simulink model "copy2"  (R2019a)
settings: Solver=FixedStepAuto  StartTime=0.0  StopTime=inf  FixedStep=0.000001  RelTol=1e-3
libraries: dspstat3 x4, simulink x1
settings Model: NumberOfSteps=16  Creator=vardhah  LastModifiedBy=vardhah
settings DataIOCC: ReturnWorkspaceOutputs=off
settings DebuggingCC: UnderSpecifiedDimensionMsg=warning  ArithmeticOperatorsInVariantConditions=warning

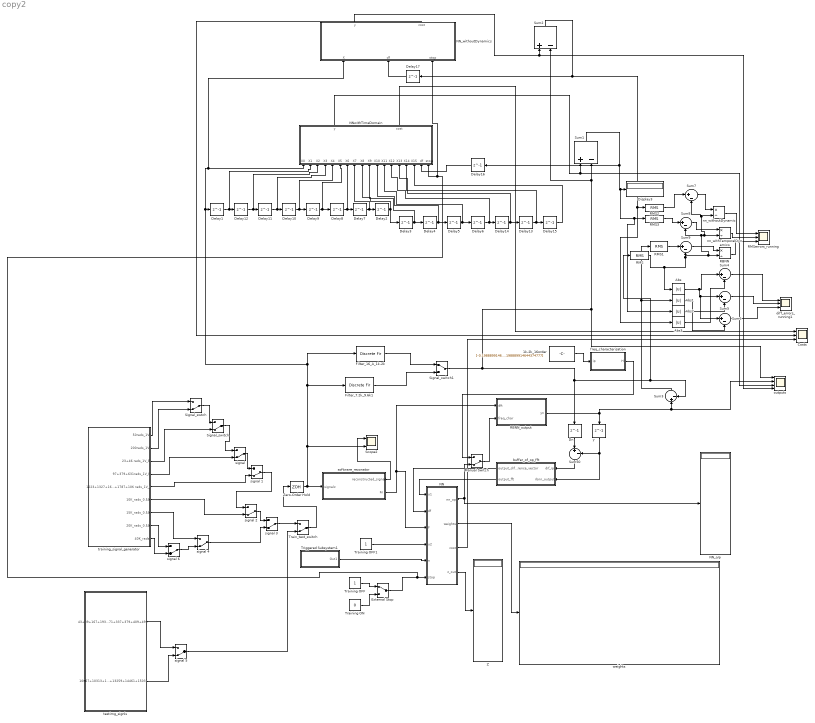
== system copy2 ==
  1k-2k_16order : Constant  Value=[-0.198889914644374777 0.0882189428518377339 0.0736891495871065116 0.0638368801789635787 0.0566372642221577294 0.0523172683654103132 0.0494565343907736044 0.048157521822162791 0.048157521822162791 0.0494565343907736044 0.0523172683654103132 0.0566372642221577294 0.0638368801789635787 0.0736891495871065116 0.0882189428518377339 -0.198889914644374777]  VectorParams1D=off
  Abs{,1..3} (4 alike) : Abs
  Costs : Scope  NumInputPorts=3
  Delay{1..17} (17 alike) : Delay  DelayLength=1  InitialCondition=0
  Display3 : Display
  Dn : Delay  DelayLength=1  InitialCondition=0
  External Stop : ManualSwitch
  Filter_16_A_1k-2k : DiscreteFir  Tag=BlockMethodSubSystem  Coefficients=[-0.198889914644374777 0.0882189428518377339 0.0736891495871065116 0.0638368801789635787 0.0566372642221577294 0.0523172683654103132 0.0494565343907736044 0.048157521822162791 0.048157521822162791 0.0494565343907736044 0.0523172683654103132 0.0566372642221577294 0.0638368801789635787 0.0736891495871065116 0.0882189428518377339 -0.198889914644374777]  InputProcessing=Columns as channels (frame based)
  Filter_7.2k_9.6k1 : DiscreteFir  Tag=BlockMethodSubSystem  Coefficients=[-0.0120785049852322399 -0.0942455273574688279 0.0101245004695954266 0.125460404555770566 0.034165372769331126 -0.1614987160724079 -0.0984930555982914957 0.150982315564688691 0.150982315564688691 -0.0984930555982914957 -0.1614987160724079 0.034165372769331126 0.125460404555770566 0.0101245004695954266 -0.0942455273574688279 -0.0120785049852322399]  InputProcessing=Columns as channels (frame based)
  Manual Switch : ManualSwitch  CurrentSetting=0  varsize=on
  NN : MATLAB Function  TreatAsAtomicUnit=on
  NN_o/p : Display
  NN_withoutDynamics : MATLAB Function  TreatAsAtomicUnit=on
  NNwithTimeDomain : MATLAB Function  TreatAsAtomicUnit=on
  RBNN : Product  Inputs=*/
  RBNN_output : MATLAB Function  TreatAsAtomicUnit=on
  RMS{,1..3} (4 alike) : dspstat3/RMS  run=on  directionMode=Each column  dimension=1  InputProcessing=Columns as channels (frame based)  reset_popup=None
  RMSerrors_running : Scope  NumInputPorts=3
  Scope2 : Scope  NumInputPorts=2
  Signal_switch : ManualSwitch  CurrentSetting=0
  Signal_switch1 : ManualSwitch
  Signal_swtch : ManualSwitch  CurrentSetting=0
  Sum1 : Sum  Inputs=+-
  Sum2 : Sum  Inputs=+-
  Sum{3..9,50} (8 alike) : Sum  Inputs=|+-
  Train_test_switch : ManualSwitch  CurrentSetting=0
  Training OFF : Constant
  Training OFF1 : Constant
  Training ON : Constant  Value=0
  Triggered Subsystem1 : Subsystem  TreatAsAtomicUnit=on
  Z : Display
  Zero-Order Hold : ZeroOrderHold  SampleTime=0.00001
  buffer_of_op_fft : MATLAB Function  TreatAsAtomicUnit=on
  diff_errors_running1 : Scope  NumInputPorts=3
  freq_characterisation : MATLAB Function  TreatAsAtomicUnit=on
  nn_withTemporalDynamics : Product  Inputs=*/
  nn_withoutDynamic : Product  Inputs=*/
  outputs : Scope  NumInputPorts=4
  signal {,1..6} (7 alike) : ManualSwitch  CurrentSetting=0
  software_rezonator : MATLAB Function  TreatAsAtomicUnit=on
  testimg_signls : Subsystem
  training_signal_generator : Subsystem
  weights : Display
  y : Delay  DelayLength=1  InitialCondition=0
  wires:
  software_rezonator/1(reconstructed_signal) -> Scope2/1
  software_rezonator/2(Fn) -> RBNN_output/1(dft), NN/3(F)
  RBNN_output/1(yn) -> Sum3/1, outputs/2, y/1
  Dn/1 -> Sum50/1
  y/1 -> buffer_of_op_fft/2(rbnn_output), Sum50/2
  Manual Switch/1 -> RBNN_output/2(freq_char)
  freq_characterisation/1(H) -> Manual Switch/1
  NN/1(nn_op) -> Manual Switch/2, NN_o/p/1
  External Stop/1 -> NN_withoutDynamics/3(stop), NNwithTimeDomain/18(stop), NN/6(stop)
  Training OFF/1 -> External Stop/1
  Training ON/1 -> External Stop/2
  NN/3(cost) -> Costs/3
  NN/2(weights) -> weights/1
  NN/4(z_out) -> Z/1
  1k-2k_16order/1 -> freq_characterisation/1(ip)
  Triggered Subsystem1/1(Out1) -> NN/5(n)
  Sum50/1 -> buffer_of_op_fft/1(dif_ip)
  buffer_of_op_fft/1(output_difference_vector) -> NN/2(df)
  buffer_of_op_fft/2(output_fft) -> NN/1(u1)
  Training OFF1/1 -> NN/4(u2)
  Signal_switch/1 -> "signal "/1
  Signal_swtch/1 -> Signal_switch/1
  "signal "/1 -> signal 1/1
  signal 1/1 -> signal 2/1
  training_signal_generator/4(97+379+631rads_1V_E) -> "signal "/2
  training_signal_generator/1(50rads_1V) -> Signal_swtch/1
  training_signal_generator/2(200rads_1V) -> Signal_swtch/2
  training_signal_generator/3(23+46 rads_1V_E) -> Signal_switch/2
  training_signal_generator/5(1223+1327+1637+1787+10K rads_1V_E) -> signal 1/2
  training_signal_generator/6(10K_rads_0.5A) -> signal 2/2
  signal 2/1 -> signal 3/1
  NNwithTimeDomain/1(y) -> outputs/3, Sum1/1
  Delay16/1 -> NNwithTimeDomain/17(df)
  Delay4/1 -> NNwithTimeDomain/11(X10), Delay5/1
  Delay6/1 -> Delay14/1, NNwithTimeDomain/13(X12)
  Delay5/1 -> NNwithTimeDomain/12(X11), Delay6/1
  NNwithTimeDomain/2(cost) -> Costs/1
  Delay2/1 -> Delay3/1, NNwithTimeDomain/9(X8)
  Delay15/1 -> NNwithTimeDomain/16(X15)
  Delay13/1 -> NNwithTimeDomain/15(X14), Delay15/1
  Delay14/1 -> NNwithTimeDomain/14(X13), Delay13/1
  Delay10/1 -> NNwithTimeDomain/5(X4), Delay9/1
  Zero-Order Hold/1 -> Scope2/2, Filter_16_A_1k-2k/1, NN_withoutDynamics/1(X), NNwithTimeDomain/1(X0), Delay1/1, Filter_7.2k_9.6k1/1, software_rezonator/1(signalz)
  Delay3/1 -> Delay4/1, NNwithTimeDomain/10(X9)
  Delay7/1 -> Delay2/1, NNwithTimeDomain/8(X7)
  Delay8/1 -> NNwithTimeDomain/7(X6), Delay7/1
  Delay1/1 -> NNwithTimeDomain/2(X1), Delay12/1
  Delay9/1 -> Delay8/1, NNwithTimeDomain/6(X5)
  Delay12/1 -> NNwithTimeDomain/3(X2), Delay11/1
  Delay11/1 -> Delay10/1, NNwithTimeDomain/4(X3)
  Sum1/1 -> Abs2/1, RMS3/1, Display3/1, Delay16/1
  NN_withoutDynamics/1(y) -> outputs/4, Sum2/1
  Delay17/1 -> NN_withoutDynamics/2(df)
  Sum2/1 -> Abs3/1, RMS2/1, Delay17/1
  NN_withoutDynamics/2(cost) -> Costs/2
  training_signal_generator/7(15K_rads_0.5A) -> signal 4/1
  signal 4/1 -> signal 3/2
  Filter_7.2k_9.6k1/1 -> Signal_switch1/2
  Filter_16_A_1k-2k/1 -> Signal_switch1/1
  Signal_switch1/1 -> Sum2/2, Sum1/2, outputs/1, RMS/1, Sum3/2, Dn/1
  nn_withoutDynamic/1 -> RMSerrors_running/1
  nn_withTemporalDynamics/1 -> RMSerrors_running/2
  RBNN/1 -> RMSerrors_running/3
  RMS/1 -> Sum7/2, nn_withoutDynamic/2, nn_withTemporalDynamics/2, Sum8/2, RBNN/2, Sum9/2, Abs/1
  Sum3/1 -> Abs1/1, RMS1/1
  Abs/1 -> Sum6/1, Sum5/1, Sum4/1
  Abs1/1 -> Sum6/2
  Abs3/1 -> Sum4/2
  Abs2/1 -> Sum5/2
  Sum4/1 -> diff_errors_running1/1
  Sum5/1 -> diff_errors_running1/2
  Sum6/1 -> diff_errors_running1/3
  RMS1/1 -> Sum9/1
  RMS3/1 -> Sum8/1
  Sum8/1 -> nn_withTemporalDynamics/1
  RMS2/1 -> Sum7/1
  Sum7/1 -> nn_withoutDynamic/1
  testimg_signls/1(43+89+167+193+229+271+337+379+409+499) -> signal 5/1
  testimg_signls/2("10067+10313+10987+11299+11491+12161+12451+13259+14461+15031 ") -> signal 5/2
  signal 3/1 -> Train_test_switch/1
  signal 5/1 -> Train_test_switch/2
  Train_test_switch/1 -> Zero-Order Hold/1
  signal 6/1 -> signal 4/2
  training_signal_generator/8(20K_rads_0.5A) -> signal 6/1
  training_signal_generator/9(40K_rads) -> signal 6/2
  Sum9/1 -> RBNN/1

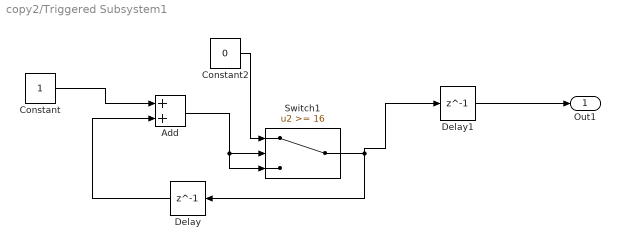
== system copy2/Triggered Subsystem1 ==
  Add : Sum
  Constant : Constant
  Constant2 : Constant  Value=0
  Delay : Delay  DelayLength=1  InitialCondition=0
  Delay1 : Delay  DelayLength=1  InitialCondition=0
  Switch1 : Switch  Threshold=16
  Out1 : Outport
  wires:
  Constant2/1 -> Switch1/1
  Constant/1 -> Add/1
  Switch1/1 -> Delay1/1, Delay/1
  Delay/1 -> Add/2
  Add/1 -> Switch1/3, Switch1/2
  Delay1/1 -> Out1/1

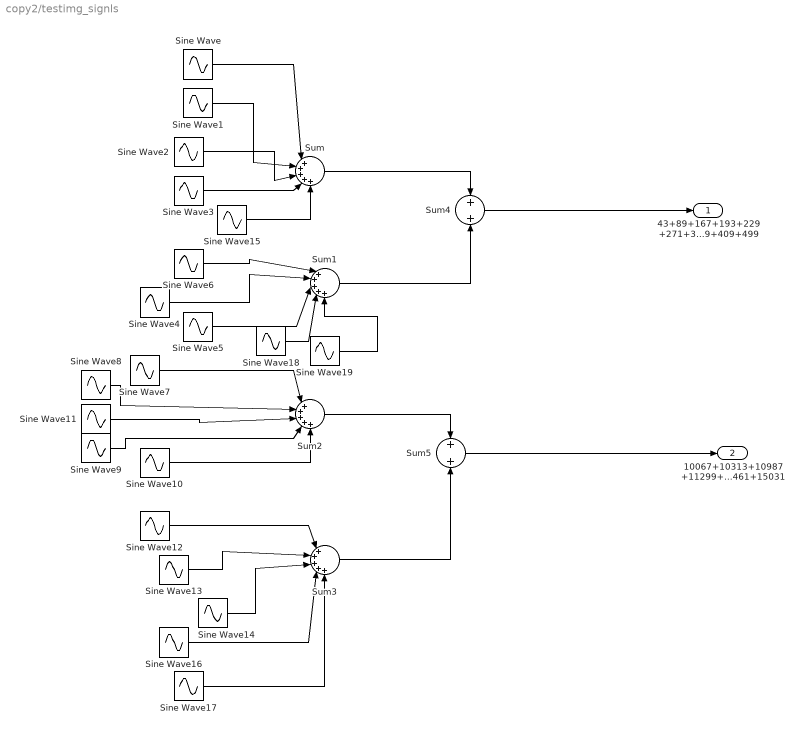
== system copy2/testimg_signls ==
  Sine Wave : Sin  Amplitude=0.1  Frequency=43  SampleTime=0
  Sine Wave1 : Sin  Amplitude=0.1  Frequency=89  SampleTime=0
  Sine Wave10 : Sin  Amplitude=0.1  Frequency=11491  SampleTime=0
  Sine Wave11 : Sin  Amplitude=0.1  Frequency=10987  SampleTime=0
  Sine Wave12 : Sin  Amplitude=0.1  Frequency=12161  SampleTime=0
  Sine Wave13 : Sin  Amplitude=0.1  Frequency=12451  SampleTime=0
  Sine Wave14 : Sin  Amplitude=0.1  Frequency=13259  SampleTime=0
  Sine Wave15 : Sin  Amplitude=0.1  Frequency=229  SampleTime=0
  Sine Wave16 : Sin  Amplitude=0.1  Frequency=14461  SampleTime=0
  Sine Wave17 : Sin  Amplitude=0.1  Frequency=15031  SampleTime=0
  Sine Wave18 : Sin  Amplitude=0.1  Frequency=409  SampleTime=0
  Sine Wave19 : Sin  Amplitude=0.1  Frequency=499  SampleTime=0
  Sine Wave2 : Sin  Amplitude=0.1  Frequency=167  SampleTime=0
  Sine Wave3 : Sin  Amplitude=0.1  Frequency=193  SampleTime=0
  Sine Wave4 : Sin  Amplitude=0.1  Frequency=337  SampleTime=0
  Sine Wave5 : Sin  Amplitude=0.1  Frequency=379  SampleTime=0
  Sine Wave6 : Sin  Amplitude=0.1  Frequency=271  SampleTime=0
  Sine Wave7 : Sin  Amplitude=0.1  Frequency=10067  SampleTime=0
  Sine Wave8 : Sin  Amplitude=0.1  Frequency=10313  SampleTime=0
  Sine Wave9 : Sin  Amplitude=0.1  Frequency=11299  SampleTime=0
  Sum{,1..3} (4 alike) : Sum  Inputs=|+++++
  Sum4 : Sum
  Sum5 : Sum
  43+89+167+193+229+271+337+379+409+499 : Outport
  "10067+10313+10987+11299+11491+12161+12451+13259+14461+15031 " : Outport  Port=2
  wires:
  Sine Wave4/1 -> Sum1/2
  Sine Wave5/1 -> Sum1/3
  Sine Wave6/1 -> Sum1/1
  Sine Wave7/1 -> Sum2/1
  Sine Wave8/1 -> Sum2/2
  Sine Wave11/1 -> Sum2/3
  Sine Wave9/1 -> Sum2/4
  Sine Wave10/1 -> Sum2/5
  Sine Wave/1 -> Sum/1
  Sine Wave1/1 -> Sum/2
  Sine Wave2/1 -> Sum/3
  Sine Wave3/1 -> Sum/4
  Sine Wave15/1 -> Sum/5
  Sine Wave17/1 -> Sum3/5
  Sine Wave16/1 -> Sum3/4
  Sine Wave14/1 -> Sum3/3
  Sine Wave13/1 -> Sum3/2
  Sine Wave12/1 -> Sum3/1
  Sine Wave18/1 -> Sum1/4
  Sine Wave19/1 -> Sum1/5
  Sum1/1 -> Sum4/2
  Sum/1 -> Sum4/1
  Sum4/1 -> 43+89+167+193+229+271+337+379+409+499/1
  Sum5/1 -> "10067+10313+10987+11299+11491+12161+12451+13259+14461+15031 "/1
  Sum2/1 -> Sum5/1
  Sum3/1 -> Sum5/2

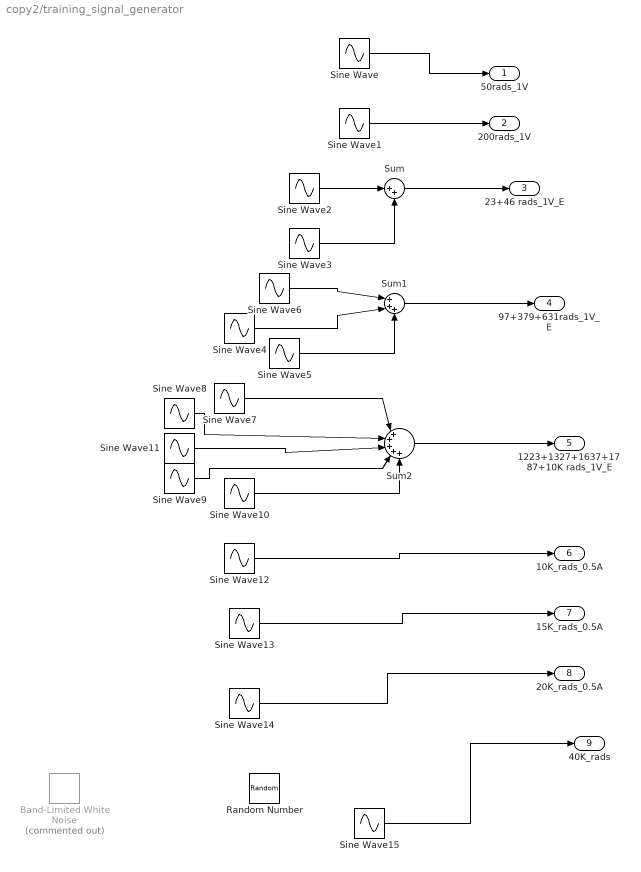
== system copy2/training_signal_generator ==
  Band-Limited White Noise : simulink/Sources/Band-Limited White Noise  Commented=on  Cov=[0.1]  Ts=0.1  seed=[23341]
  Random Number : RandomNumber  Variance=0.5  SampleTime=0.0001
  Sine Wave : Sin  Frequency=50  SampleTime=0
  Sine Wave1 : Sin  Frequency=200  SampleTime=0
  Sine Wave10 : Sin  Amplitude=0.2  Frequency=10000  SampleTime=0
  Sine Wave11 : Sin  Amplitude=0.2  Frequency=1637  SampleTime=0
  Sine Wave12 : Sin  Amplitude=0.5  Frequency=10000  SampleTime=0
  Sine Wave13 : Sin  Amplitude=0.5  Frequency=15000  SampleTime=0
  Sine Wave14 : Sin  Amplitude=0.5  Frequency=20000  SampleTime=0
  Sine Wave15 : Sin  Amplitude=0.5  Frequency=40000  SampleTime=0
  Sine Wave2 : Sin  Amplitude=0.5  Frequency=23  SampleTime=0
  Sine Wave3 : Sin  Amplitude=0.5  Frequency=46  SampleTime=0
  Sine Wave4 : Sin  Amplitude=0.33  Frequency=631  SampleTime=0
  Sine Wave5 : Sin  Amplitude=0.33  Frequency=379  SampleTime=0
  Sine Wave6 : Sin  Amplitude=0.33  Frequency=97  SampleTime=0
  Sine Wave7 : Sin  Amplitude=0.2  Frequency=1223  SampleTime=0
  Sine Wave8 : Sin  Amplitude=0.2  Frequency=1327  SampleTime=0
  Sine Wave9 : Sin  Amplitude=0.2  Frequency=1787  SampleTime=0
  Sum : Sum  Inputs=|++
  Sum1 : Sum  Inputs=|+++
  Sum2 : Sum  Inputs=|+++++
  50rads_1V : Outport
  200rads_1V : Outport  Port=2
  23+46 rads_1V_E : Outport  Port=3
  97+379+631rads_1V_E : Outport  Port=4
  1223+1327+1637+1787+10K rads_1V_E : Outport  Port=5
  10K_rads_0.5A : Outport  Port=6
  15K_rads_0.5A : Outport  Port=7
  20K_rads_0.5A : Outport  Port=8
  40K_rads : Outport  Port=9
  wires:
  Sine Wave/1 -> 50rads_1V/1
  Sine Wave1/1 -> 200rads_1V/1
  Sine Wave2/1 -> Sum/1
  Sine Wave3/1 -> Sum/2
  Sum/1 -> 23+46 rads_1V_E/1
  Sine Wave4/1 -> Sum1/2
  Sine Wave5/1 -> Sum1/3
  Sine Wave6/1 -> Sum1/1
  Sum1/1 -> 97+379+631rads_1V_E/1
  Sine Wave7/1 -> Sum2/1
  Sine Wave8/1 -> Sum2/2
  Sine Wave11/1 -> Sum2/3
  Sine Wave9/1 -> Sum2/4
  Sine Wave10/1 -> Sum2/5
  Sum2/1 -> 1223+1327+1637+1787+10K rads_1V_E/1
  Sine Wave12/1 -> 10K_rads_0.5A/1
  Sine Wave13/1 -> 15K_rads_0.5A/1
  Sine Wave14/1 -> 20K_rads_0.5A/1
  Sine Wave15/1 -> 40K_rads/1

== matlab function copy2/NN_withoutDynamics ==
  settings: sampleTime=0.125
  data: X input; df input; y output; cost output; stop input
function [y,cost] = NN_withoutDynamics(X,df,stop)

%This is a generalised code for 2 layer - multiple input-single output network.
% to alter the network (1) "change layer's size" in layer declaration below (2) the function
%input and output above and (3) Input matrix creation. (4) change inputs in
%simulink design

alpha = 0.01;

%(1)layer decalration
layer_0= 1;
layer_1= 256;
layer_2 =1;


%(2) is above in function block

%(3)parameter intialisation
v=X;

%Do not alter the code below. The below implementaion is generalised for
%multiple input and single output, 2 layer neural network. 


persistent w1 w2;
persistent a1 a2;
persistent J; 
persistent v_old; 

if isempty(a1)
    a1= zeros(layer_1,1);
end

if isempty(a2)
    a2= zeros(layer_2,1);
end


if isempty(J)
    J= 0;
end
if isempty(v_old)
    v_old= zeros(1,layer_0);
end



if isempty(w1)
       w1=randn(layer_1,layer_0);
end
if isempty(w2)
       w2=randn(layer_2,layer_1);
end

%BackProp:
if stop==0
dz2=a2.*(1-a2)*df*-1;
dw2=dz2*transpose(a1);
dz1=a1.*(1-a1)*dz2;
dw1=dz1*v;
w2=w2 + alpha*dw2;
w1=w1 + alpha*dw1;
v_old=v;
end 

%forward propogation
z1=w1*v';
a1= (1./(1+exp(-z1)));
an1=a1-0.5;
z2=w2*an1;
a2= (1./(1+exp(-z2)));
an2=a2-0.5;
cost=1/2*df^2;

%output assignment
y=an2;


end

== matlab function copy2/NN ==
  settings: sampleTime=0.01
  data: u1 input; df input; F input; u2 input; nn_op output; n input; weights output; cost output; z_out output; stop input
function [nn_op,weights,cost,z_out]  = NN(u1,df,F,u2,n,stop)

persistent w1;
persistent vy;
persistent g;
persistent itr;
persistent J;
persistent del_w;
persistent mult;
persistent memory_alloc_flag;

alpha = 0.9;
%layer declaration
input_layer = 17; 
layer_1=16;

if isempty(memory_alloc_flag)
        memory_alloc_flag = 0; 
end
if isempty(mult)
       mult=zeros(layer_1,layer_1*input_layer); 
end
if memory_alloc_flag==0
 %write memory allocation for looped code here.. 
 mult=[];
  for itr =1:layer_1
   mult=[mult;[zeros(1,(itr-1)*input_layer) ones(1,input_layer) zeros(1,(input_layer-itr-1)*input_layer)]];
 end
 memory_alloc_flag=1;
end

if isempty(del_w)
    del_w=zeros(1,272);
end

if isempty(itr)
    itr=0;
end
if isempty(J)
    J=0;
end

%gradient initialisation
if isempty(g)
    g= zeros(16,272);
   %g= rand(16,272);   
end


%prestored Vy matrix
if isempty(vy)
    vy=[0.0625000000000000,0.0625000000000000,0.0625000000000000,0.0625000000000000,0.0625000000000000,0.0625000000000000,0.0625000000000000,0.0625000000000000,0.0625000000000000,0.0625000000000000,0.0625000000000000,0.0625000000000000,0.0625000000000000,0.0625000000000000,0.0625000000000000,0.0625000000000000;0.0577424707819554,0.0441941738241592,0.0239177145228181,-1.14810637420064e-17,-0.0239177145228181,-0.0441941738241592,-0.0577424707819554,-0.0625000000000000,-0.0577424707819554,-0.0441941738241592,-0.0239177145228181,3.82702124733548e-18,0.0239177145228181,0.0441941738241592,0.0577424707819554,0.0625000000000000;0.0441941738241592,-2.67891487313484e-17,-0.0441941738241592,-0.0625000000000000,-0.0441941738241592,1.91351062366774e-17,0.0441941738241592,0.0625000000000000,0.0441941738241592,-1.14810637420064e-17,-0.0441941738241592,-0.0625000000000000,-0.0441941738241592,3.82702124733548e-18,0.0441941738241592,0.0625000000000000;0.0239177145228179,-0.0441941738241592,-0.0577424707819554,3.44431912260193e-17,0.0577424707819555,0.0441941738241592,-0.0239177145228182,-0.0625000000000000,-0.0239177145228181,0.0441941738241592,0.0577424707819554,-1.14810637420064e-17,-0.0577424707819554,-0.0441941738241592,0.0239177145228181,0.0625000000000000;-1.68427621172548e-16,-0.0625000000000000,-6.12710262471544e-17,0.0625000000000000,-1.53119536183206e-16,-0.0625000000000000,3.44431912260193e-17,0.0625000000000000,-2.67891487313484e-17,-0.0625000000000000,1.91351062366774e-17,0.0625000000000000,-1.14810637420064e-17,-0.0625000000000000,3.82702124733548e-18,0.0625000000000000;-0.0239177145228182,-0.0441941738241591,0.0577424707819554,-1.68427621172548e-16,-0.0577424707819554,0.0441941738241592,0.0239177145228181,-0.0625000000000000,0.0239177145228182,0.0441941738241592,-0.0577424707819554,1.91351062366774e-17,0.0577424707819554,-0.0441941738241592,-0.0239177145228181,0.0625000000000000;-0.0441941738241596,-3.06548562684706e-17,0.0441941738241593,-0.0625000000000000,0.0441941738241594,-1.68427621172548e-16,-0.0441941738241592,0.0625000000000000,-0.0441941738241592,3.44431912260193e-17,0.0441941738241592,-0.0625000000000000,0.0441941738241592,-1.14810637420064e-17,-0.0441941738241592,0.0625000000000000;-0.0577424707819556,0.0441941738241594,-0.0239177145228178,-3.06548562684706e-17,0.0239177145228179,-0.0441941738241591,0.0577424707819554,-0.0625000000000000,0.0577424707819555,-0.0441941738241592,0.0239177145228182,-2.67891487313484e-17,-0.0239177145228181,0.0441941738241592,-0.0577424707819554,0.0625000000000000;-0.0625000000000000,0.0625000000000000,-0.0625000000000000,0.0625000000000000,-0.0625000000000000,0.0625000000000000,-0.0625000000000000,0.0625000000000000,-0.0625000000000000,0.0625000000000000,-0.0625000000000000,0.0625000000000000,-0.0625000000000000,0.0625000000000000,-0.0625000000000000,0.0625000000000000;-0.0239177145228184,0.0441941738241592,-0.0577424707819555,0.0625000000000000,-0.0577424707819553,0.0441941738241592,-0.0239177145228180,-6.88863824520386e-17,0.0239177145228181,-0.0441941738241593,0.0577424707819554,-0.0625000000000000,0.0577424707819554,-0.0441941738241592,0.0239177145228181,0;-0.0441941738241594,0.0625000000000000,-0.0441941738241593,-3.36855242345096e-16,0.0441941738241595,-0.0625000000000000,0.0441941738241592,7.65404249467096e-17,-0.0441941738241593,0.0625000000000000,-0.0441941738241592,-3.82702124733548e-17,0.0441941738241593,-0.0625000000000000,0.0441941738241592,0;-0.0577424707819556,0.0441941738241592,0.0239177145228178,-0.0625000000000000,0.0239177145228177,0.0441941738241592,-0.0577424707819555,-3.06239072366412e-16,0.0577424707819554,-0.0441941738241592,-0.0239177145228181,0.0625000000000000,-0.0239177145228181,-0.0441941738241593,0.0577424707819554,0;-0.0625000000000000,6.13097125369412e-17,0.0625000000000000,1.37772764904077e-16,-0.0625000000000000,-3.36855242345096e-16,0.0625000000000000,9.18485099360515e-17,-0.0625000000000000,-6.88863824520386e-17,0.0625000000000000,4.59242549680257e-17,-0.0625000000000000,-2.29621274840129e-17,0.0625000000000000,0;-0.0577424707819553,-0.0441941738241594,0.0239177145228181,0.0625000000000000,0.0239177145228186,-0.0441941738241590,-0.0577424707819555,1.22542052494309e-16,0.0577424707819554,0.0441941738241593,-0.0239177145228180,-0.0625000000000000,-0.0239177145228182,0.0441941738241592,0.0577424707819554,0;-0.0441941738241587,-0.0625000000000000,-0.0441941738241588,6.13097125369412e-17,0.0441941738241588,0.0625000000000000,0.0441941738241592,1.07156594925393e-16,-0.0441941738241590,-0.0625000000000000,-0.0441941738241593,-5.35782974626967e-17,0.0441941738241592,0.0625000000000000,0.0441941738241592,0;-0.0239177145228178,-0.0441941738241593,-0.0577424707819556,-0.0625000000000000,-0.0577424707819556,-0.0441941738241594,-0.0239177145228184,-3.36855242345096e-16,0.0239177145228181,0.0441941738241592,0.0577424707819554,0.0625000000000000,0.0577424707819554,0.0441941738241593,0.0239177145228182,0;0,0,0,0,0,0,0,0,0,0,0,0,0,0,0,0];
end



%input initialisation
x_in = [real(u1(1)) real(u1(2)) real(u1(3)) real(u1(4)) real(u1(5)) real(u1(6)) real(u1(7)) real(u1(8)) real(u1(9)) imag(u1(1)) imag(u1(2)) imag(u1(3)) imag(u1(4)) imag(u1(5)) imag(u1(6)) imag(u1(7))];

%parameter intialisation 
v=transpose([x_in u2]);
if isempty(w1)
       w1=randn(input_layer,layer_1)*0.1;
end


%F=transpose([real(X0) 2*(real(X1)*cos(pi*1*n/8)-imag(X1)*sin(pi*1*n/8)) 2*(real(X2)*cos(pi*2*n/8)-imag(X2)*sin(pi*2*n/8)) 2*(real(X3)*cos(pi*3*n/8)-imag(X3)*sin(pi*3*n/8)) 2*(real(X4)*cos(pi*4*n/8)-imag(X4)*sin(pi*4*n/8)) 2*(real(X5)*cos(pi*5*n/8)-imag(X5)*sin(pi*5*n/8)) 2*(real(X6)*cos(pi*6*n/8)-imag(X6)*sin(pi*6*n/8)) 2*(real(X7)*cos(pi*7*n/8)-imag(X7)*sin(pi*7*n/8)) -1^n*real(X8) -2*(imag(X9)*cos(pi*9*n/8)+real(X9)*sin(pi*9*n/8)) -2*(imag(X10)*cos(pi*10*n/8)+real(X10)*sin(pi*10*n/8)) -2*(imag(X11)*cos(pi*11*n/8)+real(X11)*sin(pi*11*n/8)) -2*(imag(X12)*cos(pi*12*n/8)+real(X12)*sin(pi*12*n/8)) -2*(imag(X13)*cos(pi*13*n/8)+real(X13)*sin(pi*13*n/8)) -2*(imag(X14)*cos(pi*14*n/8)+real(X14)*sin(pi*14*n/8)) -2*(imag(X15)*cos(pi*15*n/8)+real(X15)*sin(pi*15*n/8))]); 
%u_out=v;


%forward propogation
z=w1'*v ;
z_out=z;
a=(1./(1+exp(-z)));
an=(a-0.5);

%calculation of Nv:
dz_a=a.*(1-a);                  
Nv=w1'.* repmat(dz_a,1, size(w1,1));

%calculation of aD
aD=transpose(F)*Nv*vy;
A=[aD;eye(15) zeros(15,1)];
B=[transpose(F) ; zeros(15,16)];   
dw1=v*transpose(dz_a);

%added to vectorise the implementation
Expanded_dw1=repmat(transpose(dw1),1,size(dw1,2));
Nw=Expanded_dw1.*mult; 
g=A*g+B*Nw;



if n==15 && stop==0
    del_w =alpha*df*1*g/16 ;
    del_w_reshaped= reshape(del_w,[17,16]);
    w1=w1+ del_w_reshaped;
    itr=itr+1;
    
end
J= 1/32*sum(df.^2,'all');
cost=J;
weights=w1;


nn_op=an;


end

== matlab function copy2/buffer_of_op_fft ==
  data: output_difference_vector output size=[1,16]; output_fft output size=[1,16]; dif_ip input; rbnn_output input
function [output_difference_vector,output_fft] = difBuffer(dif_ip,rbnn_output)                      

 sz=16;                       % size of the dft 
 
 persistent a;
 persistent b;
 if isempty(b)
  b= zeros(1,sz);
 end
 if isempty(a)
  a= zeros(1,sz);
 end
 
 
  a= circshift(a,1);
  a(1)=dif_ip;
  b= circshift(b,1);
  b(1)=rbnn_output;

 output_difference_vector=a; 
 output_fft=1/sz*fft(b); 
end

== matlab function copy2/freq_characterisation ==
  data: ip input; H output
function H  = freq_character(ip)                      

dft_of_ip=fft(ip); 
size_dft=size(dft_of_ip,2)/2;
H =transpose([real(dft_of_ip(1:size_dft+1)) imag(dft_of_ip(2:size_dft))]);

end

== matlab function copy2/NNwithTimeDomain ==
  settings: sampleTime=0.125
  data: X0 input; X1 input; X2 input; X3 input; X4 input; X5 input; X6 input; X7 input; X8 input; X9 input; X10 input; X11 input; X12 input; X13 input; X14 input; X15 input; df input; y output; cost output; stop input
function [y,cost] = NN(X0,X1,X2,X3,X4,X5,X6,X7,X8,X9,X10,X11,X12,X13,X14,X15,df,stop)

%This is a generalised code for 2 layer - multiple input-single output network.
% to alter the network (1) "change layer's size" in layer declaration below (2) the function
%input and output above and (3) Input matrix creation. (4) change inputs in
%simulink design

alpha = 0.03;

%(1)layer decalration
layer_0= 16;
layer_1= 16;
layer_2 =1;


%(2) is above in function block

%(3)parameter intialisation
v=[X0 X1 X2 X3 X4 X5 X6 X7 X8 X9 X10 X11 X12 X13 X14 X15];

%Do not alter the code below. The below implementaion is generalised for
%multiple input and single output, 2 layer neural network. 


persistent w1 w2;
persistent a1 a2;
persistent J; 
persistent v_old; 

if isempty(a1)
    a1= zeros(layer_1,1);
end

if isempty(a2)
    a2= zeros(layer_2,1);
end


if isempty(J)
    J= 0;
end
if isempty(v_old)
    v_old= zeros(1,layer_0);
end



if isempty(w1)
       w1=randn(layer_1,layer_0);
end
if isempty(w2)
       w2=randn(layer_2,layer_1);
end

%BackProp:
if stop==0
dz2=a2.*(1-a2)*df*-1;
dw2=dz2*transpose(a1);
dz1=a1.*(1-a1)*dz2;
dw1=dz1*v;
w2=w2 + alpha*dw2;
w1=w1 + alpha*dw1;
v_old=v;
end 

%forward propogation
z1=w1*v';
a1= (1./(1+exp(-z1)));
an1=a1-0.5;
z2=w2*an1;
a2= (1./(1+exp(-z2)));
an2=a2-0.5;
cost=1/2*df^2;

%output assignment
y=an2;


end

== matlab function copy2/software_rezonator ==
  data: signalz input; reconstructed_signal output; Fn output size=16
function [reconstructed_signal,Fn]   = rezonator(signalz)

persistent numberofrezonator;
persistent g c bfr_rezo_sm aft_delay dft_out;
persistent out signal_dif;
persistent n;
persistent memory_alloc_flag;


%assign the number of rezonator here. For configuring it for higher order
%rezonator  we need to change (1) 'numberofrezonaotor' variable
if isempty(numberofrezonator)
        numberofrezonator = 16;   %here 16 parallel rezonators
end

%Initialisation of memory allocations/variables ====> 
if isempty(memory_alloc_flag)
        memory_alloc_flag = 0; 
end
if isempty(g)
       g=zeros(numberofrezonator,numberofrezonator,'like',0i); 
end
if isempty(c)
       c=zeros(numberofrezonator,numberofrezonator,'like',0i); 
end
if memory_alloc_flag==0
 for i=0:numberofrezonator-1
  for j= 0:numberofrezonator-1
   g(i+1,j+1)=1/numberofrezonator*(exp(-1i*2*pi*i*j/numberofrezonator));
   c(i+1,j+1)=(exp(1i*2*pi*i*j/numberofrezonator));
  end 
 end
 memory_alloc_flag=1;
end


%Initialisation of variables  =====> 
if isempty(n)
        n = 0;   
end 
if isempty(out)
  out=0+0i;
end
if isempty(signal_dif)
  signal_dif=0+0i;
end
if isempty(bfr_rezo_sm)
  bfr_rezo_sm=repmat(0+0i,numberofrezonator,1);
end
if isempty(aft_delay)
  aft_delay=repmat(0+0i,numberofrezonator,1);
end
if isempty(dft_out)
  dft_out=repmat(0+0i,numberofrezonator,1);
end

%creating cycle of rotation for selection of correct column of g & c.
cycle=mod(n,numberofrezonator);

%resonator core -----------------------------> 
dft_out=c(:,cycle+1).*aft_delay;
out= sum(dft_out,1);
signal_dif=signalz-out;
bfr_rezo_sm=g(:,cycle+1).*signal_dif;

%counting the counter
n=n+1;

% output assignment ------------------>
reconstructed_signal=out;
dft=aft_delay; 
N=size(dft,1);
a=1:1:N/2-1;
b=N/2+1:1:N-1;
dft_trans=transpose(dft);
Fn=transpose([real(dft_trans(1)) 2*(real(dft_trans(2:N/2)).*cos(2*pi*a*n/N)-imag(dft_trans(2:N/2)).*sin(2*pi*a*n/N)) -1^n*real(dft_trans(N/2+1)) -2*(imag(dft_trans(N/2+2:N)).*cos(2*pi*b*n/N)+real(dft_trans(N/2+2:N)).*sin(2*pi*b*n/N))]);
%--------output assignment over----------<

%final updation of buffer ------>>>>>>>>>>>>
aft_delay= aft_delay+bfr_rezo_sm; 
end

== matlab function copy2/RBNN_output ==
  data: dft input; yn output; freq_char input
function yn = fcn(dft,freq_char)
yn=transpose(freq_char)*dft;
end
